simulink model "gait_testing"  (R2024a)
settings: Solver=ode23t  StartTime=0.0  StopTime=8  RelTol=1e-3  AbsTol=1e-3  EnableMultiTasking=on
model workspace (MAT data in the model file):
  A = 0.4
  Length_torso : Simulink.Parameter (value not decoded)
  Lower_limbs : Simulink.Parameter (value not decoded)
  Upper_limbs : Simulink.Parameter (value not decoded)
  Width_torso : Simulink.Parameter (value not decoded)
  f = 1.5
  r_foot : Simulink.Parameter (value not decoded)
  t_leg : Simulink.Parameter (value not decoded)
symbols that are objects in the model workspace (value not decoded): Length_torso, Lower_limbs, t_leg, Upper_limbs, Width_torso
undefined symbols (not defined in the file): P0x, P0z, P1x, P1z, P2x, P2z, X, Y, Z
libraries: sm_lib x88, functionAngles x16, functionAnglesSide x16, nesl_utility x15
(part 4 of 10)

== system gait_testing/Gait Selector/Walk Back Gait - Bezier Curves ==
  t : Inport
  tdur : Inport  Port=2
  change? : Inport  Port=3
  Action Port : ActionPort  InitializeStates=reset  ActionPortLabel=case [ 3 ]:
  Bus Creator : BusCreator  Inputs=12
  Constant{,1..3} (4 alike) : Constant  Value=0
  MATLAB Function : MATLAB Function  TreatAsAtomicUnit=on
  Mod4 : Math  Operator=mod
  Plane Movement : Subsystem
  Plane Movement1 : Subsystem
  Plane Movement2 : Subsystem
  Plane Movement3 : Subsystem
  Plane Movement4 : Subsystem
  Sin-Movement : Subsystem
  Stop when change : Subsystem
  delay and stop when change : Subsystem  mask{delay=0.5}
  delay and stop when change1 : Subsystem  mask{delay=0.25}
  delay and stop when change2 : Subsystem  mask{delay=0.75}
  q : Outport
  wires:
  Constant2/1 -> Bus Creator/12  "sBRs"
  Constant3/1 -> Bus Creator/9  "sBLs"
  Constant1/1 -> Bus Creator/6  "sFRs"
  Constant/1 -> Bus Creator/3  "sFLs"
  Plane Movement3/1(hip) -> Bus Creator/10  "sBR"
  Plane Movement3/2(knee) -> Bus Creator/11  "kBR"
  Plane Movement2/1(hip) -> Bus Creator/7  "sBL"
  Plane Movement2/2(knee) -> Bus Creator/8  "kBL"
  Plane Movement1/2(knee) -> Bus Creator/5  "kFR"
  Plane Movement4/2(knee) -> Bus Creator/2  "kFL"
  Plane Movement1/1(hip) -> Bus Creator/4  "sFR"
  Plane Movement4/1(hip) -> Bus Creator/1  "sFL"
  Bus Creator/1 -> q/1
  Mod4/1 -> Stop when change/3(t_leg)  "t"
  Stop when change/1(t_out) -> Plane Movement4/1(t)
  delay and stop when change2/1(t_leg) -> Plane Movement3/1(t)
  delay and stop when change1/1(t_leg) -> Plane Movement2/1(t)
  MATLAB Function/1(activationTime) -> Stop when change/5(activation time), delay and stop when change2/1(activationTime), delay and stop when change1/1(activationTime), delay and stop when change/1(activationTime)
  delay and stop when change/1(t_leg) -> Plane Movement1/1(t)
  change?/1 -> Stop when change/1(change?), delay and stop when change2/4(Change?), delay and stop when change1/4(Change?), delay and stop when change/4(Change?)
  tdur/1 -> Plane Movement1/2(tdur), delay and stop when change/3(tdur), Plane Movement3/2(tdur), delay and stop when change2/3(tdur), Plane Movement2/2(tdur), delay and stop when change1/3(tdur), Mod4/2, Stop when change/4(tdur), Plane Movement4/2(tdur)
  t/1 -> delay and stop when change2/2(t), delay and stop when change1/2(t), delay and stop when change/2(t), MATLAB Function/1(u), Stop when change/2(t), Mod4/1

== system gait_testing/Gait Selector/Walk Gait - Bezier Curves ==
  t : Inport
  tdur : Inport  Port=2
  Change? : Inport  Port=3
  Action Port : ActionPort  InitializeStates=reset  ActionPortLabel=case [ 1 ]:
  Bus Creator : BusCreator  Inputs=12
  Constant{,1..3} (4 alike) : Constant  Value=0
  MATLAB Function : MATLAB Function  TreatAsAtomicUnit=on
  Mod4 : Math  Operator=mod
  Plane Movement : Subsystem
  Plane Movement1 : Subsystem
  Plane Movement2 : Subsystem
  Plane Movement3 : Subsystem
  Plane Movement4 : Subsystem
  Scope : Scope  NumInputPorts=2
  Sin-Movement : Subsystem
  Stop when change : Subsystem
  delay and stop when change : Subsystem  mask{delay=0.5}
  delay and stop when change1 : Subsystem  mask{delay=0.75}
  delay and stop when change2 : Subsystem  mask{delay=0.25}
  q : Outport
  wires:
  Constant2/1 -> Bus Creator/12  "sBRs"
  Constant3/1 -> Bus Creator/9  "sBLs"
  Constant1/1 -> Bus Creator/6  "sFRs"
  Constant/1 -> Bus Creator/3  "sFLs"
  Mod4/1 -> Stop when change/3(t_leg)  "t"
  tdur/1 -> delay and stop when change2/3(tdur), Plane Movement3/2(tdur), delay and stop when change1/3(tdur), Plane Movement2/2(tdur), Plane Movement1/2(tdur), delay and stop when change/3(tdur), Mod4/2, Stop when change/4(tdur), Plane Movement4/2(tdur)
  t/1 -> Mod4/1, Stop when change/2(t), MATLAB Function/1(u), delay and stop when change2/2(t), delay and stop when change1/2(t), delay and stop when change/2(t)
  Plane Movement3/1(hip) -> Bus Creator/10  "sBR"
  Plane Movement3/2(knee) -> Bus Creator/11  "kBR"
  Plane Movement2/1(hip) -> Bus Creator/7  "sBL"
  Plane Movement2/2(knee) -> Bus Creator/8  "kBL"
  Plane Movement1/2(knee) -> Bus Creator/5  "kFR"
  Plane Movement4/2(knee) -> Scope/1, Bus Creator/2  "kFL"
  Plane Movement1/1(hip) -> Bus Creator/4  "sFR"
  Plane Movement4/1(hip) -> Scope/2, Bus Creator/1  "sFL"
  Bus Creator/1 -> q/1
  MATLAB Function/1(activationTime) -> Stop when change/5(activation time), delay and stop when change2/1(activationTime), delay and stop when change1/1(activationTime), delay and stop when change/1(activationTime)
  delay and stop when change/1(t_leg) -> Plane Movement1/1(t)
  Change?/1 -> delay and stop when change/4(Change?), delay and stop when change1/4(Change?), delay and stop when change2/4(Change?), Stop when change/1(change?)
  Stop when change/1(t_out) -> Plane Movement4/1(t)
  delay and stop when change1/1(t_leg) -> Plane Movement2/1(t)
  delay and stop when change2/1(t_leg) -> Plane Movement3/1(t)

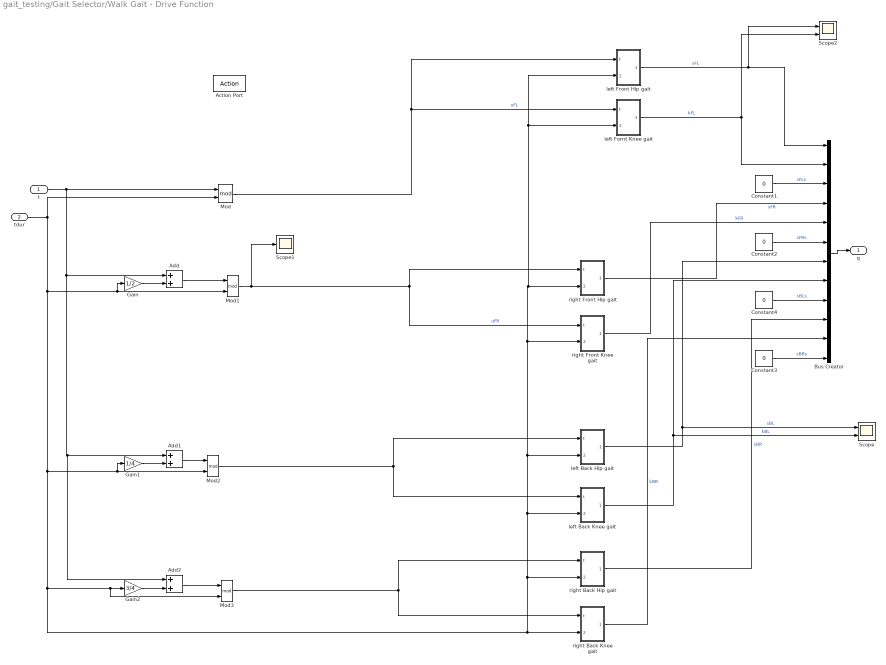
== system gait_testing/Gait Selector/Walk Gait - Drive Function ==
  t : Inport
  tdur : Inport  Port=2
  Action Port : ActionPort  InitializeStates=reset
  Add : Sum
  Add1 : Sum
  Add2 : Sum
  Bus Creator : BusCreator  Inputs=12
  Constant{1..4} (4 alike) : Constant  Value=0
  Gain : Gain  Gain=1/2
  Gain1 : Gain  Gain=1/4
  Gain2 : Gain  Gain=3/4
  Mod{,1..3} (4 alike) : Math  Operator=mod
  Scope : Scope  NumInputPorts=2
  Scope1 : Scope
  Scope2 : Scope  NumInputPorts=2
  left Back Hip gait : Subsystem
  left Back Knee gait : Subsystem
  left Fornt Knee gait : Subsystem
  left Front Hip gait : Subsystem
  right Back Hip gait : Subsystem
  right Back Knee gait : Subsystem
  right Front Hip gait : Subsystem
  right Front Knee gait : Subsystem
  q : Outport
  wires:
  Bus Creator/1 -> q/1
  left Front Hip gait/1(Out1) -> Scope2/1, Bus Creator/1  "sFL"
  right Front Hip gait/1(Out1) -> Bus Creator/4  "sFR"
  left Fornt Knee gait/1(Out1) -> Scope2/2, Bus Creator/2  "kFL"
  right Front Knee gait/1(Out1) -> Bus Creator/5  "kFR"
  Mod/1 -> left Front Hip gait/1(t), left Fornt Knee gait/1(t)  "uFL"
  Mod1/1 -> Scope1/1, right Front Hip gait/1(t), right Front Knee gait/1(t)  "uFR"
  left Back Knee gait/1(Out1) -> Scope/2, Bus Creator/8  "kBL"
  left Back Hip gait/1(Out1) -> Scope/1, Bus Creator/7  "sBL"
  right Back Knee gait/1(Out1) -> Bus Creator/11  "kBR"
  right Back Hip gait/1(Out1) -> Bus Creator/10  "sBR"
  Mod2/1 -> left Back Hip gait/1(t), left Back Knee gait/1(t)
  Mod3/1 -> right Back Knee gait/1(t), right Back Hip gait/1(t)
  t/1 -> Mod/1, Add2/1, Add1/1, Add/1
  Gain2/1 -> Add2/2
  tdur/1 -> Mod/2, left Back Knee gait/2(tdur), left Back Hip gait/2(tdur), right Front Knee gait/2(tdur), right Front Hip gait/2(tdur), left Front Hip gait/2(tdur), left Fornt Knee gait/2(tdur), right Back Hip gait/2(tdur), right Back Knee gait/2(tdur), Gain2/1, Mod3/2, Mod2/2, Gain1/1, Gain/1, Mod1/2
  Add1/1 -> Mod2/1
  Add/1 -> Mod1/1
  Gain/1 -> Add/2
  Gain1/1 -> Add1/2
  Add2/1 -> Mod3/1
  Constant1/1 -> Bus Creator/3  "sFLs"
  Constant3/1 -> Bus Creator/12  "sBRs"
  Constant4/1 -> Bus Creator/9  "sBLs"
  Constant2/1 -> Bus Creator/6  "sFRs"

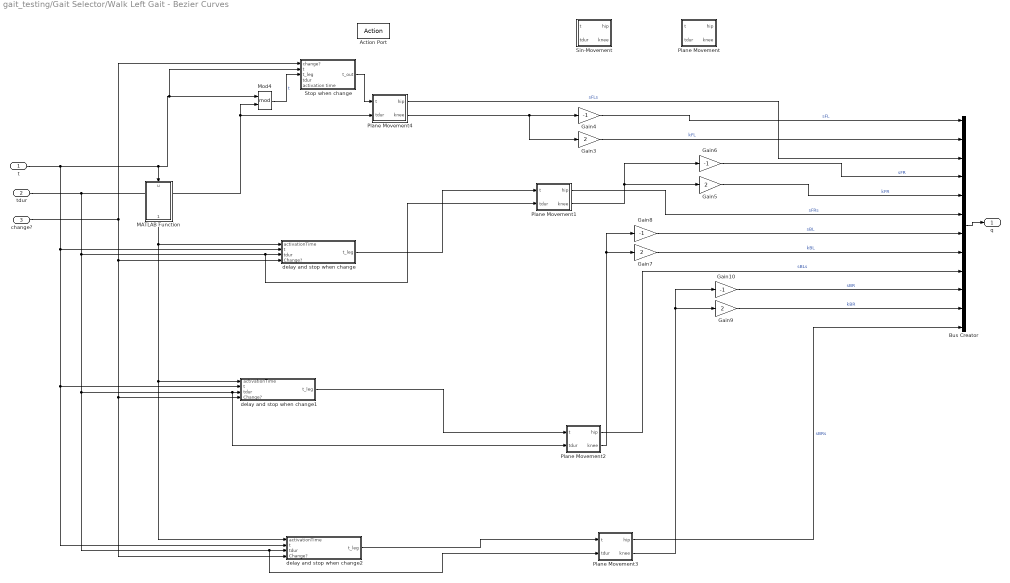
== system gait_testing/Gait Selector/Walk Left Gait - Bezier Curves ==
  t : Inport
  tdur : Inport  Port=2
  change? : Inport  Port=3
  Action Port : ActionPort  InitializeStates=reset  ActionPortLabel=case [ 4 ]:
  Bus Creator : BusCreator  Inputs=12
  Gain{4,6,8,10} (4 alike) : Gain  Gain=-1
  Gain{3,5,7,9} (4 alike) : Gain  Gain=2
  MATLAB Function : MATLAB Function  TreatAsAtomicUnit=on
  Mod4 : Math  Operator=mod
  Plane Movement : Subsystem
  Plane Movement1 : Subsystem
  Plane Movement2 : Subsystem
  Plane Movement3 : Subsystem
  Plane Movement4 : Subsystem
  Sin-Movement : Subsystem
  Stop when change : Subsystem
  delay and stop when change : Subsystem  mask{delay=0.5}
  delay and stop when change1 : Subsystem  mask{delay=0.25}
  delay and stop when change2 : Subsystem  mask{delay=0.75}
  q : Outport
  wires:
  Bus Creator/1 -> q/1
  Plane Movement4/1(hip) -> Bus Creator/3  "sFLs"
  Plane Movement1/1(hip) -> Bus Creator/6  "sFRs"
  Plane Movement4/2(knee) -> Gain3/1, Gain4/1
  Plane Movement1/2(knee) -> Gain6/1, Gain5/1
  Plane Movement2/2(knee) -> Gain7/1, Gain8/1
  Plane Movement2/1(hip) -> Bus Creator/9  "sBLs"
  Plane Movement3/2(knee) -> Gain10/1, Gain9/1
  Plane Movement3/1(hip) -> Bus Creator/12  "sBRs"
  Mod4/1 -> Stop when change/3(t_leg)  "t"
  Gain4/1 -> Bus Creator/1  "sFL"
  Gain5/1 -> Bus Creator/5  "kFR"
  Gain6/1 -> Bus Creator/4  "sFR"
  Gain7/1 -> Bus Creator/8  "kBL"
  Gain8/1 -> Bus Creator/7  "sBL"
  Gain9/1 -> Bus Creator/11  "kBR"
  Gain10/1 -> Bus Creator/10  "sBR"
  Gain3/1 -> Bus Creator/2  "kFL"
  Stop when change/1(t_out) -> Plane Movement4/1(t)
  delay and stop when change2/1(t_leg) -> Plane Movement3/1(t)
  delay and stop when change1/1(t_leg) -> Plane Movement2/1(t)
  delay and stop when change/1(t_leg) -> Plane Movement1/1(t)
  t/1 -> delay and stop when change2/2(t), delay and stop when change1/2(t), delay and stop when change/2(t), Stop when change/2(t), Mod4/1, MATLAB Function/1(u)
  change?/1 -> delay and stop when change2/4(Change?), delay and stop when change1/4(Change?), delay and stop when change/4(Change?), Stop when change/1(change?)
  tdur/1 -> Plane Movement1/2(tdur), delay and stop when change/3(tdur), Plane Movement3/2(tdur), delay and stop when change2/3(tdur), Plane Movement2/2(tdur), delay and stop when change1/3(tdur), Plane Movement4/2(tdur), Mod4/2
  MATLAB Function/1(activationTime) -> delay and stop when change/1(activationTime), delay and stop when change2/1(activationTime), delay and stop when change1/1(activationTime)

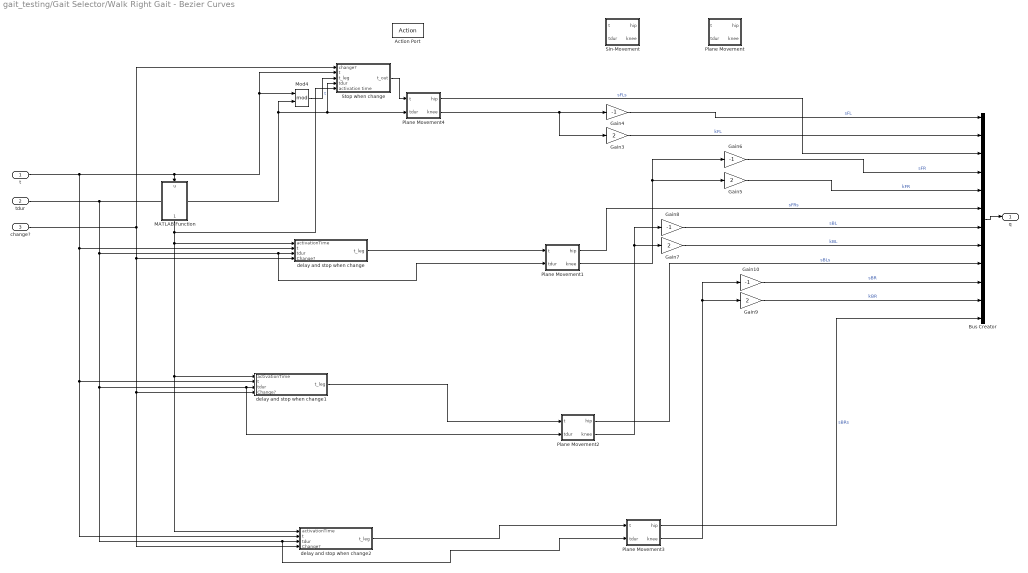
== system gait_testing/Gait Selector/Walk Right Gait - Bezier Curves ==
  t : Inport
  tdur : Inport  Port=2
  change? : Inport  Port=3
  Action Port : ActionPort  InitializeStates=reset  ActionPortLabel=case [ 5 ]:
  Bus Creator : BusCreator  Inputs=12
  Gain{4,6,8,10} (4 alike) : Gain  Gain=-1
  Gain{3,5,7,9} (4 alike) : Gain  Gain=2
  MATLAB Function : MATLAB Function  TreatAsAtomicUnit=on
  Mod4 : Math  Operator=mod
  Plane Movement : Subsystem
  Plane Movement1 : Subsystem
  Plane Movement2 : Subsystem
  Plane Movement3 : Subsystem
  Plane Movement4 : Subsystem
  Sin-Movement : Subsystem
  Stop when change : Subsystem
  delay and stop when change : Subsystem  mask{delay=0.5}
  delay and stop when change1 : Subsystem  mask{delay=0.25}
  delay and stop when change2 : Subsystem  mask{delay=0.75}
  q : Outport
  wires:
  Gain3/1 -> Bus Creator/2  "kFL"
  Gain10/1 -> Bus Creator/10  "sBR"
  Gain9/1 -> Bus Creator/11  "kBR"
  Gain8/1 -> Bus Creator/7  "sBL"
  Gain7/1 -> Bus Creator/8  "kBL"
  Gain6/1 -> Bus Creator/4  "sFR"
  Gain5/1 -> Bus Creator/5  "kFR"
  Gain4/1 -> Bus Creator/1  "sFL"
  Mod4/1 -> Stop when change/3(t_leg)  "t"
  Plane Movement3/1(hip) -> Bus Creator/12  "sBRs"
  Plane Movement3/2(knee) -> Gain9/1, Gain10/1
  Plane Movement2/1(hip) -> Bus Creator/9  "sBLs"
  Plane Movement2/2(knee) -> Gain8/1, Gain7/1
  Plane Movement1/2(knee) -> Gain5/1, Gain6/1
  Plane Movement4/2(knee) -> Gain4/1, Gain3/1
  Plane Movement1/1(hip) -> Bus Creator/6  "sFRs"
  Plane Movement4/1(hip) -> Bus Creator/3  "sFLs"
  Bus Creator/1 -> q/1
  Stop when change/1(t_out) -> Plane Movement4/1(t)
  delay and stop when change2/1(t_leg) -> Plane Movement3/1(t)
  delay and stop when change1/1(t_leg) -> Plane Movement2/1(t)
  delay and stop when change/1(t_leg) -> Plane Movement1/1(t)
  t/1 -> delay and stop when change2/2(t), delay and stop when change1/2(t), delay and stop when change/2(t), Stop when change/2(t), Mod4/1, MATLAB Function/1(u)
  change?/1 -> delay and stop when change2/4(Change?), delay and stop when change1/4(Change?), delay and stop when change/4(Change?), Stop when change/1(change?)
  tdur/1 -> Plane Movement1/2(tdur), delay and stop when change/3(tdur), Plane Movement3/2(tdur), delay and stop when change2/3(tdur), Plane Movement2/2(tdur), delay and stop when change1/3(tdur), Mod4/2, Stop when change/4(tdur), Plane Movement4/2(tdur)
  MATLAB Function/1(activationTime) -> Stop when change/5(activation time), delay and stop when change/1(activationTime), delay and stop when change2/1(activationTime), delay and stop when change1/1(activationTime)

== system gait_testing/Gait Selector/Stand Still/Plane Movement ==
  t : Inport
  tdur : Inport  Port=2
  Constant : Constant  Value=P0x
  Constant1 : Constant  Value=P0z
  Constant2 : Constant  Value=P1z
  Constant3 : Constant  Value=P1x
  Constant4 : Constant  Value=P2x
  Constant5 : Constant  Value=P2z
  Constant6 : Constant  Value=P3x
  Constant7 : Constant  Value=P3z
  Gain : Gain  Gain=180/pi
  Gain1 : Gain  Gain=-180/pi
  Length lower Limb : Constant  Value=Lower_limbs
  Length upper Limb : Constant  Value=Upper_limbs
  MATLAB Function1 : MATLAB Function  TreatAsAtomicUnit=on
  MATLAB Function2 : MATLAB Function  TreatAsAtomicUnit=on
  Scope : Scope  NumInputPorts=2
  Subsystem1 : Subsystem  Commented=on
  hip : Outport
  knee : Outport  Port=2
  wires:
  MATLAB Function2/2(y) -> MATLAB Function1/2(y), Scope/2
  MATLAB Function2/1(x) -> Scope/1, MATLAB Function1/1(x)
  MATLAB Function1/2(theta2) -> Gain1/1  "knee"
  tdur/1 -> MATLAB Function2/2(Tdur)
  MATLAB Function1/1(theta1) -> Gain/1  "hip"
  t/1 -> MATLAB Function2/1(t)
  Length upper Limb/1 -> MATLAB Function1/3(L1)
  Length lower Limb/1 -> MATLAB Function1/4(L2)
  Gain1/1 -> knee/1
  Gain/1 -> hip/1
  Constant/1 -> MATLAB Function2/3(P0x)
  Constant1/1 -> MATLAB Function2/4(P0z)
  Constant3/1 -> MATLAB Function2/5(P1x)
  Constant2/1 -> MATLAB Function2/6(P1z)
  Constant4/1 -> MATLAB Function2/7(P2x)
  Constant5/1 -> MATLAB Function2/8(P2z)
  Constant6/1 -> MATLAB Function2/9(P3x)
  Constant7/1 -> MATLAB Function2/10(P3z)

== system gait_testing/Gait Selector/Stand Still/Plane Movement1 ==
  t : Inport
  tdur : Inport  Port=2
  Constant : Constant  Value=P3x
  Constant1 : Constant  Value=P3z
  Gain : Gain  Gain=180/pi
  Gain1 : Gain  Gain=-180/pi
  Length lower Limb : Constant  Value=Lower_limbs
  Length upper Limb : Constant  Value=Upper_limbs
  MATLAB : functionAngles/MATLAB  SystemSampleTime=-1  VariantActivationTime=update diagram  AllowFlexibleInterface=on  Latency=0  AutoFrameSizeCalculation=off
  Subsystem1 : Subsystem  Commented=on
  hip : Outport
  knee : Outport  Port=2
  wires:
  MATLAB/2 -> Gain1/1  "knee"
  tdur/1 -> ?
  MATLAB/1 -> Gain/1  "hip"
  t/1 -> ?
  Length upper Limb/1 -> MATLAB/3
  Length lower Limb/1 -> MATLAB/4
  Gain1/1 -> knee/1
  Gain/1 -> hip/1
  Constant/1 -> MATLAB/1
  Constant1/1 -> MATLAB/2

== system gait_testing/Gait Selector/Stand Still/Plane Movement2 ==
  t : Inport
  tdur : Inport  Port=2
  Constant : Constant  Value=P3x
  Constant1 : Constant  Value=P3z
  Gain : Gain  Gain=180/pi
  Gain1 : Gain  Gain=-180/pi
  Length lower Limb : Constant  Value=Lower_limbs
  Length upper Limb : Constant  Value=Upper_limbs
  MATLAB : functionAngles/MATLAB  SystemSampleTime=-1  VariantActivationTime=update diagram  AllowFlexibleInterface=on  Latency=0  AutoFrameSizeCalculation=off
  Subsystem1 : Subsystem  Commented=on
  hip : Outport
  knee : Outport  Port=2
  wires:
  Constant1/1 -> MATLAB/2
  Constant/1 -> MATLAB/1
  Gain/1 -> hip/1
  Gain1/1 -> knee/1
  Length lower Limb/1 -> MATLAB/4
  Length upper Limb/1 -> MATLAB/3
  t/1 -> ?
  MATLAB/1 -> Gain/1  "hip"
  tdur/1 -> ?
  MATLAB/2 -> Gain1/1  "knee"

== system gait_testing/Gait Selector/Stand Still/Plane Movement3 ==
  t : Inport
  tdur : Inport  Port=2
  Constant : Constant  Value=P3x
  Constant1 : Constant  Value=P3z
  Gain : Gain  Gain=180/pi
  Gain1 : Gain  Gain=-180/pi
  Length lower Limb : Constant  Value=Lower_limbs
  Length upper Limb : Constant  Value=Upper_limbs
  MATLAB : functionAngles/MATLAB  SystemSampleTime=-1  VariantActivationTime=update diagram  AllowFlexibleInterface=on  Latency=0  AutoFrameSizeCalculation=off
  Subsystem1 : Subsystem  Commented=on
  hip : Outport
  knee : Outport  Port=2
  wires:
  MATLAB/2 -> Gain1/1  "knee"
  tdur/1 -> ?
  MATLAB/1 -> Gain/1  "hip"
  t/1 -> ?
  Length upper Limb/1 -> MATLAB/3
  Length lower Limb/1 -> MATLAB/4
  Gain1/1 -> knee/1
  Gain/1 -> hip/1
  Constant/1 -> MATLAB/1
  Constant1/1 -> MATLAB/2

== system gait_testing/Gait Selector/Stand Still/Plane Movement4 ==
  t : Inport
  tdur : Inport  Port=2
  Constant : Constant  Value=P3x
  Constant1 : Constant  Value=P3z
  Gain : Gain  Gain=180/pi
  Gain1 : Gain  Gain=-180/pi
  Length lower Limb : Constant  Value=Lower_limbs
  Length upper Limb : Constant  Value=Upper_limbs
  MATLAB : functionAngles/MATLAB  SystemSampleTime=-1  VariantActivationTime=update diagram  AllowFlexibleInterface=on  Latency=0  AutoFrameSizeCalculation=off
  Subsystem1 : Subsystem  Commented=on
  hip : Outport
  knee : Outport  Port=2
  wires:
  Constant1/1 -> MATLAB/2
  Constant/1 -> MATLAB/1
  Gain/1 -> hip/1
  Gain1/1 -> knee/1
  Length lower Limb/1 -> MATLAB/4
  Length upper Limb/1 -> MATLAB/3
  t/1 -> ?
  MATLAB/1 -> Gain/1  "hip"
  tdur/1 -> ?
  MATLAB/2 -> Gain1/1  "knee"

== system gait_testing/Gait Selector/Stand Still/Sin-Movement ==
  t : Inport
  tdur : Inport  Port=2
  Constant : Constant  Value=P0x
  Constant1 : Constant  Value=P0z
  Constant2 : Constant  Value=P1z
  Constant3 : Constant  Value=P1x
  Constant4 : Constant  Value=P2x
  Constant5 : Constant  Value=P2z
  Constant6 : Constant  Value=P3x
  Constant7 : Constant  Value=P3z
  Gain : Gain  Gain=180/pi
  Gain1 : Gain  Gain=-180/pi
  Length lower Limb : Constant  Value=Lower_limbs
  Length upper Limb : Constant  Value=Upper_limbs
  MATLAB Function : MATLAB Function  TreatAsAtomicUnit=on
  MATLAB Function1 : MATLAB Function  TreatAsAtomicUnit=on
  Scope : Scope  NumInputPorts=2
  Subsystem1 : Subsystem  Commented=on
  hip : Outport
  knee : Outport  Port=2
  wires:
  MATLAB Function/2(y) -> MATLAB Function1/2(y), Scope/2
  MATLAB Function/1(x) -> MATLAB Function1/1(x), Scope/1
  MATLAB Function1/2(theta2) -> Gain1/1  "knee"
  tdur/1 -> MATLAB Function/2(Tdur)
  MATLAB Function1/1(theta1) -> Gain/1  "hip"
  t/1 -> MATLAB Function/1(t)
  Length upper Limb/1 -> MATLAB Function1/3(L1)
  Length lower Limb/1 -> MATLAB Function1/4(L2)
  Gain1/1 -> knee/1
  Gain/1 -> hip/1
  Constant/1 -> MATLAB Function/3(P0x)
  Constant1/1 -> MATLAB Function/4(P0z)
  Constant3/1 -> MATLAB Function/5(P1x)
  Constant2/1 -> MATLAB Function/6(P1z)
  Constant4/1 -> MATLAB Function/7(P2x)
  Constant5/1 -> MATLAB Function/8(P2z)
  Constant6/1 -> MATLAB Function/9(P3x)
  Constant7/1 -> MATLAB Function/10(P3z)

== system gait_testing/Gait Selector/Trot Gait - Bezier Curves/Plane Movement ==
  t : Inport
  tdur : Inport  Port=2
  Constant : Constant  Value=P0x
  Constant1 : Constant  Value=P0z
  Constant2 : Constant  Value=P1z
  Constant3 : Constant  Value=P1x
  Constant4 : Constant  Value=P2x
  Constant5 : Constant  Value=P2z
  Constant6 : Constant  Value=P3x
  Constant7 : Constant  Value=P3z
  Gain : Gain  Gain=180/pi
  Gain1 : Gain  Gain=-180/pi
  Length lower Limb : Constant  Value=Lower_limbs
  Length upper Limb : Constant  Value=Upper_limbs
  MATLAB Function1 : MATLAB Function  TreatAsAtomicUnit=on
  MATLAB Function2 : MATLAB Function  TreatAsAtomicUnit=on
  Scope : Scope  NumInputPorts=2
  Subsystem1 : Subsystem  Commented=on
  hip : Outport
  knee : Outport  Port=2
  wires:
  MATLAB Function2/2(y) -> MATLAB Function1/2(y), Scope/2
  MATLAB Function2/1(x) -> Scope/1, MATLAB Function1/1(x)
  MATLAB Function1/2(theta2) -> Gain1/1  "knee"
  tdur/1 -> MATLAB Function2/2(Tdur)
  MATLAB Function1/1(theta1) -> Gain/1  "hip"
  t/1 -> MATLAB Function2/1(t)
  Length upper Limb/1 -> MATLAB Function1/3(L1)
  Length lower Limb/1 -> MATLAB Function1/4(L2)
  Gain1/1 -> knee/1
  Gain/1 -> hip/1
  Constant/1 -> MATLAB Function2/3(P0x)
  Constant1/1 -> MATLAB Function2/4(P0z)
  Constant3/1 -> MATLAB Function2/5(P1x)
  Constant2/1 -> MATLAB Function2/6(P1z)
  Constant4/1 -> MATLAB Function2/7(P2x)
  Constant5/1 -> MATLAB Function2/8(P2z)
  Constant6/1 -> MATLAB Function2/9(P3x)
  Constant7/1 -> MATLAB Function2/10(P3z)

== system gait_testing/Gait Selector/Trot Gait - Bezier Curves/Plane Movement1 ==
  t : Inport
  tdur : Inport  Port=2
  Constant : Constant  Value=P0x
  Constant1 : Constant  Value=P0z
  Constant2 : Constant  Value=P1z
  Constant3 : Constant  Value=P1x
  Constant4 : Constant  Value=P2x
  Constant5 : Constant  Value=P2z
  Constant6 : Constant  Value=P3x
  Constant7 : Constant  Value=P3z
  Gain : Gain  Gain=180/pi
  Gain1 : Gain  Gain=-180/pi
  Length lower Limb : Constant  Value=Lower_limbs
  Length upper Limb : Constant  Value=Upper_limbs
  MATLAB : functionAngles/MATLAB  SystemSampleTime=-1  VariantActivationTime=update diagram  AllowFlexibleInterface=on  Latency=0  AutoFrameSizeCalculation=off
  MATLAB Function2 : MATLAB Function  TreatAsAtomicUnit=on
  Scope : Scope  NumInputPorts=2
  Subsystem1 : Subsystem  Commented=on
  hip : Outport
  knee : Outport  Port=2
  wires:
  Constant7/1 -> MATLAB Function2/10(P3z)
  Constant6/1 -> MATLAB Function2/9(P3x)
  Constant5/1 -> MATLAB Function2/8(P2z)
  Constant4/1 -> MATLAB Function2/7(P2x)
  Constant2/1 -> MATLAB Function2/6(P1z)
  Constant3/1 -> MATLAB Function2/5(P1x)
  Constant1/1 -> MATLAB Function2/4(P0z)
  Constant/1 -> MATLAB Function2/3(P0x)
  Gain/1 -> hip/1
  Gain1/1 -> knee/1
  Length lower Limb/1 -> MATLAB/4
  Length upper Limb/1 -> MATLAB/3
  t/1 -> MATLAB Function2/1(t)
  MATLAB/1 -> Gain/1  "hip"
  tdur/1 -> MATLAB Function2/2(Tdur)
  MATLAB/2 -> Gain1/1  "knee"
  MATLAB Function2/1(x) -> MATLAB/1, Scope/1
  MATLAB Function2/2(y) -> MATLAB/2, Scope/2

== system gait_testing/Gait Selector/Trot Gait - Bezier Curves/Plane Movement2 ==
  t : Inport
  tdur : Inport  Port=2
  Constant : Constant  Value=P0x
  Constant1 : Constant  Value=P0z
  Constant2 : Constant  Value=P1z
  Constant3 : Constant  Value=P1x
  Constant4 : Constant  Value=P2x
  Constant5 : Constant  Value=P2z
  Constant6 : Constant  Value=P3x
  Constant7 : Constant  Value=P3z
  Gain : Gain  Gain=180/pi
  Gain1 : Gain  Gain=-180/pi
  Length lower Limb : Constant  Value=Lower_limbs
  Length upper Limb : Constant  Value=Upper_limbs
  MATLAB : functionAngles/MATLAB  SystemSampleTime=-1  VariantActivationTime=update diagram  AllowFlexibleInterface=on  Latency=0  AutoFrameSizeCalculation=off
  MATLAB Function2 : MATLAB Function  TreatAsAtomicUnit=on
  Scope : Scope  NumInputPorts=2
  Subsystem1 : Subsystem  Commented=on
  hip : Outport
  knee : Outport  Port=2
  wires:
  Constant7/1 -> MATLAB Function2/10(P3z)
  Constant6/1 -> MATLAB Function2/9(P3x)
  Constant5/1 -> MATLAB Function2/8(P2z)
  Constant4/1 -> MATLAB Function2/7(P2x)
  Constant2/1 -> MATLAB Function2/6(P1z)
  Constant3/1 -> MATLAB Function2/5(P1x)
  Constant1/1 -> MATLAB Function2/4(P0z)
  Constant/1 -> MATLAB Function2/3(P0x)
  Gain/1 -> hip/1
  Gain1/1 -> knee/1
  Length lower Limb/1 -> MATLAB/4
  Length upper Limb/1 -> MATLAB/3
  t/1 -> MATLAB Function2/1(t)
  MATLAB/1 -> Gain/1  "hip"
  tdur/1 -> MATLAB Function2/2(Tdur)
  MATLAB/2 -> Gain1/1  "knee"
  MATLAB Function2/1(x) -> MATLAB/1, Scope/1
  MATLAB Function2/2(y) -> MATLAB/2, Scope/2

== system gait_testing/Gait Selector/Trot Gait - Bezier Curves/Plane Movement3 ==
  t : Inport
  tdur : Inport  Port=2
  Constant : Constant  Value=P0x
  Constant1 : Constant  Value=P0z
  Constant2 : Constant  Value=P1z
  Constant3 : Constant  Value=P1x
  Constant4 : Constant  Value=P2x
  Constant5 : Constant  Value=P2z
  Constant6 : Constant  Value=P3x
  Constant7 : Constant  Value=P3z
  Gain : Gain  Gain=180/pi
  Gain1 : Gain  Gain=-180/pi
  Length lower Limb : Constant  Value=Lower_limbs
  Length upper Limb : Constant  Value=Upper_limbs
  MATLAB : functionAngles/MATLAB  SystemSampleTime=-1  VariantActivationTime=update diagram  AllowFlexibleInterface=on  Latency=0  AutoFrameSizeCalculation=off
  MATLAB Function2 : MATLAB Function  TreatAsAtomicUnit=on
  Scope : Scope  NumInputPorts=2
  Subsystem1 : Subsystem  Commented=on
  hip : Outport
  knee : Outport  Port=2
  wires:
  MATLAB Function2/2(y) -> MATLAB/2, Scope/2
  MATLAB Function2/1(x) -> MATLAB/1, Scope/1
  MATLAB/2 -> Gain1/1  "knee"
  tdur/1 -> MATLAB Function2/2(Tdur)
  MATLAB/1 -> Gain/1  "hip"
  t/1 -> MATLAB Function2/1(t)
  Length upper Limb/1 -> MATLAB/3
  Length lower Limb/1 -> MATLAB/4
  Gain1/1 -> knee/1
  Gain/1 -> hip/1
  Constant/1 -> MATLAB Function2/3(P0x)
  Constant1/1 -> MATLAB Function2/4(P0z)
  Constant3/1 -> MATLAB Function2/5(P1x)
  Constant2/1 -> MATLAB Function2/6(P1z)
  Constant4/1 -> MATLAB Function2/7(P2x)
  Constant5/1 -> MATLAB Function2/8(P2z)
  Constant6/1 -> MATLAB Function2/9(P3x)
  Constant7/1 -> MATLAB Function2/10(P3z)

== system gait_testing/Gait Selector/Trot Gait - Bezier Curves/Plane Movement4 ==
  t : Inport
  tdur : Inport  Port=2
  Constant : Constant  Value=P0x
  Constant1 : Constant  Value=P0z
  Constant2 : Constant  Value=P1z
  Constant3 : Constant  Value=P1x
  Constant4 : Constant  Value=P2x
  Constant5 : Constant  Value=P2z
  Constant6 : Constant  Value=P3x
  Constant7 : Constant  Value=P3z
  Gain : Gain  Gain=180/pi
  Gain1 : Gain  Gain=-180/pi
  Length lower Limb : Constant  Value=Lower_limbs
  Length upper Limb : Constant  Value=Upper_limbs
  MATLAB : functionAngles/MATLAB  SystemSampleTime=-1  VariantActivationTime=update diagram  AllowFlexibleInterface=on  Latency=0  AutoFrameSizeCalculation=off
  MATLAB Function2 : MATLAB Function  TreatAsAtomicUnit=on
  Scope : Scope  NumInputPorts=2
  Subsystem1 : Subsystem  Commented=on
  hip : Outport
  knee : Outport  Port=2
  wires:
  Constant7/1 -> MATLAB Function2/10(P3z)
  Constant6/1 -> MATLAB Function2/9(P3x)
  Constant5/1 -> MATLAB Function2/8(P2z)
  Constant4/1 -> MATLAB Function2/7(P2x)
  Constant2/1 -> MATLAB Function2/6(P1z)
  Constant3/1 -> MATLAB Function2/5(P1x)
  Constant1/1 -> MATLAB Function2/4(P0z)
  Constant/1 -> MATLAB Function2/3(P0x)
  Gain/1 -> hip/1
  Gain1/1 -> knee/1
  Length lower Limb/1 -> MATLAB/4
  Length upper Limb/1 -> MATLAB/3
  t/1 -> MATLAB Function2/1(t)
  MATLAB/1 -> Gain/1  "hip"
  tdur/1 -> MATLAB Function2/2(Tdur)
  MATLAB/2 -> Gain1/1  "knee"
  MATLAB Function2/1(x) -> MATLAB/1, Scope/1
  MATLAB Function2/2(y) -> MATLAB/2, Scope/2

== system gait_testing/Gait Selector/Trot Gait - Bezier Curves/Sin-Movement ==
  t : Inport
  tdur : Inport  Port=2
  Constant : Constant  Value=P0x
  Constant1 : Constant  Value=P0z
  Constant2 : Constant  Value=P1z
  Constant3 : Constant  Value=P1x
  Constant4 : Constant  Value=P2x
  Constant5 : Constant  Value=P2z
  Constant6 : Constant  Value=P3x
  Constant7 : Constant  Value=P3z
  Gain : Gain  Gain=180/pi
  Gain1 : Gain  Gain=-180/pi
  Length lower Limb : Constant  Value=Lower_limbs
  Length upper Limb : Constant  Value=Upper_limbs
  MATLAB Function : MATLAB Function  TreatAsAtomicUnit=on
  MATLAB Function1 : MATLAB Function  TreatAsAtomicUnit=on
  Scope : Scope  NumInputPorts=2
  Subsystem1 : Subsystem  Commented=on
  hip : Outport
  knee : Outport  Port=2
  wires:
  MATLAB Function/2(y) -> MATLAB Function1/2(y), Scope/2
  MATLAB Function/1(x) -> MATLAB Function1/1(x), Scope/1
  MATLAB Function1/2(theta2) -> Gain1/1  "knee"
  tdur/1 -> MATLAB Function/2(Tdur)
  MATLAB Function1/1(theta1) -> Gain/1  "hip"
  t/1 -> MATLAB Function/1(t)
  Length upper Limb/1 -> MATLAB Function1/3(L1)
  Length lower Limb/1 -> MATLAB Function1/4(L2)
  Gain1/1 -> knee/1
  Gain/1 -> hip/1
  Constant/1 -> MATLAB Function/3(P0x)
  Constant1/1 -> MATLAB Function/4(P0z)
  Constant3/1 -> MATLAB Function/5(P1x)
  Constant2/1 -> MATLAB Function/6(P1z)
  Constant4/1 -> MATLAB Function/7(P2x)
  Constant5/1 -> MATLAB Function/8(P2z)
  Constant6/1 -> MATLAB Function/9(P3x)
  Constant7/1 -> MATLAB Function/10(P3z)

== system gait_testing/Gait Selector/Trot Gait - Bezier Curves/Stop when change ==
  change? : Inport
  t : Inport  Port=2
  t_leg : Inport  Port=3
  tdur : Inport  Port=4
  activation time : Inport  Port=5
  AND : Logic  IconShape=distinctive  AllPortsSameDT=off  OutDataTypeStr=boolean
  Add : Sum  Inputs=+-
  Add2 : Sum  Inputs=+-
  Constant1 : Constant  Value=0
  Constant2 : Constant  Value=0
  OR : Logic  Operator=OR  IconShape=distinctive  AllPortsSameDT=off  OutDataTypeStr=boolean
  Relational Operator : RelationalOperator  Operator=<  OutDataTypeStr=boolean  RndMeth=Simplest  InputSameDT=off
  Relational Operator1 : RelationalOperator  Operator=<=  OutDataTypeStr=boolean  RndMeth=Simplest  InputSameDT=off
  Relational Operator2 : RelationalOperator  Operator===  OutDataTypeStr=boolean  RndMeth=Simplest  InputSameDT=off
  Relational Operator3 : RelationalOperator  Operator=>  OutDataTypeStr=boolean  RndMeth=Simplest  InputSameDT=off
  Switch : Switch  Criteria=u2 > Threshold  SaturateOnIntegerOverflow=off  InputSameDT=off
  Switch Case1 : SwitchCase  ShowDefaultCase=off
  Switch1 : Switch  Criteria=u2 > Threshold  SaturateOnIntegerOverflow=off  InputSameDT=off
  Triggered Subsystem : Subsystem  TreatAsAtomicUnit=on
  Unit Delay : UnitDelay  SampleTime=-1  HasFrameUpgradeWarning=on
  t_out : Outport
  wires:
  t_leg/1 -> Switch/3, Switch1/3, Unit Delay/1, Relational Operator/1
  Add2/1 -> Relational Operator1/1
  change?/1 -> Switch Case1/1
  Switch Case1/1 -> Triggered Subsystem/Action
  AND/1 -> Switch1/2
  Unit Delay/1 -> Relational Operator/2
  Switch1/1 -> Relational Operator2/1, Switch/1
  Relational Operator1/1 -> AND/1
  Constant2/1 -> Relational Operator2/2
  Triggered Subsystem/1(Change Time) -> Add2/2
  Relational Operator/1 -> OR/1
  tdur/1 -> Relational Operator1/2
  Relational Operator2/1 -> OR/2
  OR/1 -> AND/2
  Constant1/1 -> Switch1/1
  t/1 -> Add2/1, Add/1, Triggered Subsystem/1(t)
  Relational Operator3/1 -> Switch/2
  Switch/1 -> t_out/1
  Add/1 -> Relational Operator3/1
  activation time/1 -> Add/2

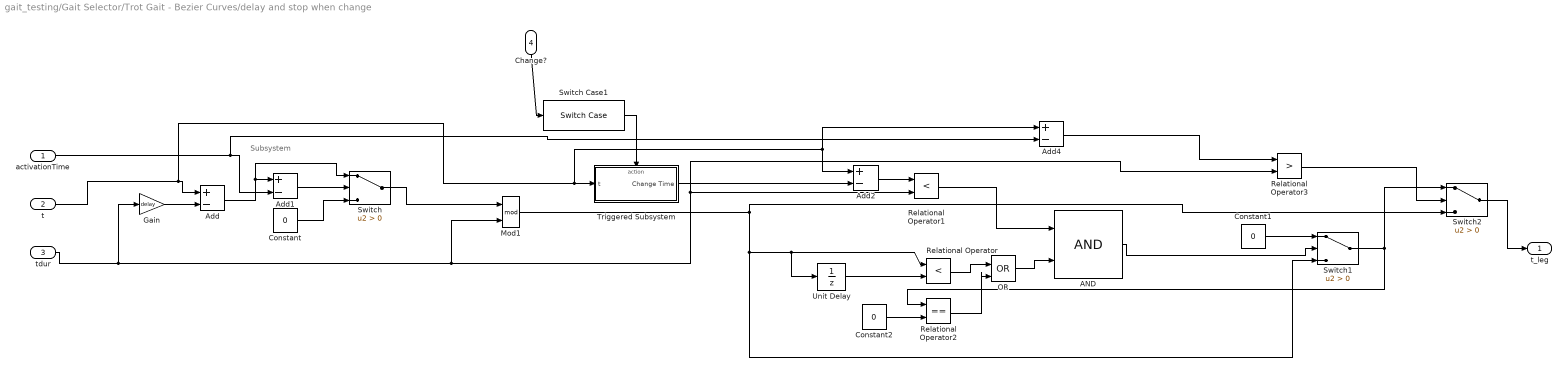
== system gait_testing/Gait Selector/Trot Gait - Bezier Curves/delay and stop when change ==
  note: Subsystem
  activationTime : Inport
  t : Inport  Port=2
  tdur : Inport  Port=3
  Change? : Inport  Port=4
  AND : Logic  IconShape=distinctive  AllPortsSameDT=off  OutDataTypeStr=boolean
  Add{,1..2,4} (4 alike) : Sum  Inputs=+-
  Constant : Constant  Value=0
  Constant1 : Constant  Value=0
  Constant2 : Constant  Value=0
  Gain : Gain  Gain=delay
  Mod1 : Math  Operator=mod
  OR : Logic  Operator=OR  IconShape=distinctive  AllPortsSameDT=off  OutDataTypeStr=boolean
  Relational Operator : RelationalOperator  Operator=<  OutDataTypeStr=boolean  RndMeth=Simplest  InputSameDT=off
  Relational Operator1 : RelationalOperator  Operator=<  OutDataTypeStr=boolean  RndMeth=Simplest  InputSameDT=off
  Relational Operator2 : RelationalOperator  Operator===  OutDataTypeStr=boolean  RndMeth=Simplest  InputSameDT=off
  Relational Operator3 : RelationalOperator  Operator=>  OutDataTypeStr=boolean  RndMeth=Simplest  InputSameDT=off
  Switch : Switch  Criteria=u2 > Threshold  SaturateOnIntegerOverflow=off  InputSameDT=off
  Switch Case1 : SwitchCase  ShowDefaultCase=off
  Switch1 : Switch  Criteria=u2 > Threshold  SaturateOnIntegerOverflow=off  InputSameDT=off
  Switch2 : Switch  Criteria=u2 > Threshold  SaturateOnIntegerOverflow=off  InputSameDT=off
  Triggered Subsystem : Subsystem  TreatAsAtomicUnit=on
  Unit Delay : UnitDelay  SampleTime=-1  HasFrameUpgradeWarning=on
  t_leg : Outport
  wires:
  Switch/1 -> Mod1/1
  Gain/1 -> Add/2
  t/1 -> Add2/1, Add4/1, Triggered Subsystem/1(t), Add/1
  Constant/1 -> Switch/3
  Add1/1 -> Switch/2
  activationTime/1 -> Add4/2, Add1/2
  Add/1 -> Switch/1, Add1/1
  Switch Case1/1 -> Triggered Subsystem/Action
  Relational Operator1/1 -> AND/1
  Constant1/1 -> Switch1/1
  Relational Operator/1 -> OR/1
  Change?/1 -> Switch Case1/1
  Unit Delay/1 -> Relational Operator/2
  AND/1 -> Switch1/2
  Switch1/1 -> Switch2/1, Relational Operator2/1
  Mod1/1 -> Switch2/3, Switch1/3, Unit Delay/1, Relational Operator/1
  Triggered Subsystem/1(Change Time) -> Add2/2
  Add2/1 -> Relational Operator1/1
  Relational Operator2/1 -> OR/2
  Constant2/1 -> Relational Operator2/2
  OR/1 -> AND/2
  Switch2/1 -> t_leg/1
  Relational Operator3/1 -> Switch2/2
  tdur/1 -> Gain/1, Mod1/2, Relational Operator3/2, Relational Operator1/2
  Add4/1 -> Relational Operator3/1

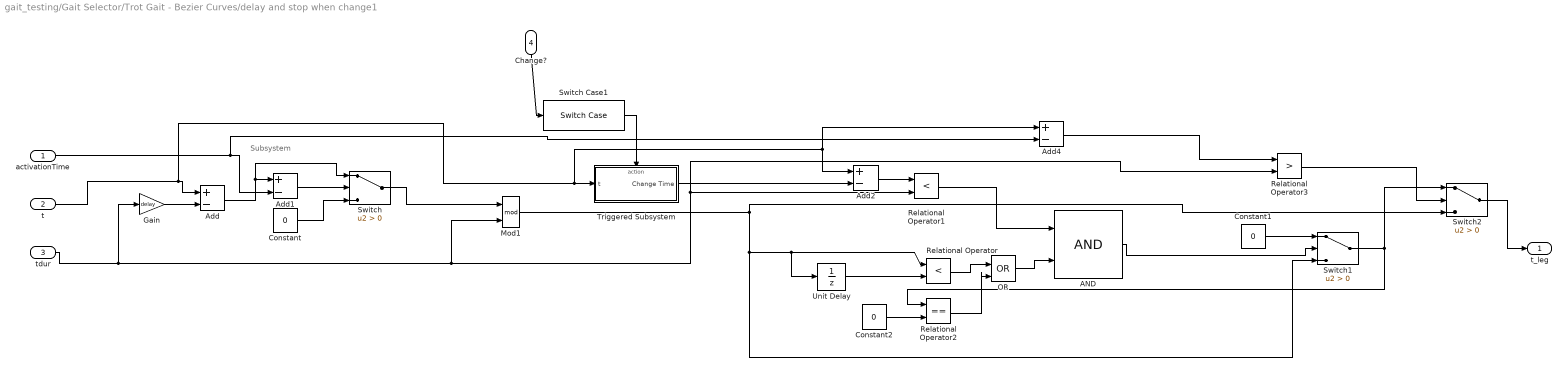
== system gait_testing/Gait Selector/Trot Gait - Bezier Curves/delay and stop when change1 ==
  note: Subsystem
  activationTime : Inport
  t : Inport  Port=2
  tdur : Inport  Port=3
  Change? : Inport  Port=4
  AND : Logic  IconShape=distinctive  AllPortsSameDT=off  OutDataTypeStr=boolean
  Add{,1..2,4} (4 alike) : Sum  Inputs=+-
  Constant : Constant  Value=0
  Constant1 : Constant  Value=0
  Constant2 : Constant  Value=0
  Gain : Gain  Gain=delay
  Mod1 : Math  Operator=mod
  OR : Logic  Operator=OR  IconShape=distinctive  AllPortsSameDT=off  OutDataTypeStr=boolean
  Relational Operator : RelationalOperator  Operator=<  OutDataTypeStr=boolean  RndMeth=Simplest  InputSameDT=off
  Relational Operator1 : RelationalOperator  Operator=<  OutDataTypeStr=boolean  RndMeth=Simplest  InputSameDT=off
  Relational Operator2 : RelationalOperator  Operator===  OutDataTypeStr=boolean  RndMeth=Simplest  InputSameDT=off
  Relational Operator3 : RelationalOperator  Operator=>  OutDataTypeStr=boolean  RndMeth=Simplest  InputSameDT=off
  Switch : Switch  Criteria=u2 > Threshold  SaturateOnIntegerOverflow=off  InputSameDT=off
  Switch Case1 : SwitchCase  ShowDefaultCase=off
  Switch1 : Switch  Criteria=u2 > Threshold  SaturateOnIntegerOverflow=off  InputSameDT=off
  Switch2 : Switch  Criteria=u2 > Threshold  SaturateOnIntegerOverflow=off  InputSameDT=off
  Triggered Subsystem : Subsystem  TreatAsAtomicUnit=on
  Unit Delay : UnitDelay  SampleTime=-1  HasFrameUpgradeWarning=on
  t_leg : Outport
  wires:
  Switch/1 -> Mod1/1
  Gain/1 -> Add/2
  t/1 -> Add2/1, Add4/1, Triggered Subsystem/1(t), Add/1
  Constant/1 -> Switch/3
  Add1/1 -> Switch/2
  activationTime/1 -> Add4/2, Add1/2
  Add/1 -> Switch/1, Add1/1
  Switch Case1/1 -> Triggered Subsystem/Action
  Relational Operator1/1 -> AND/1
  Constant1/1 -> Switch1/1
  Relational Operator/1 -> OR/1
  Change?/1 -> Switch Case1/1
  Unit Delay/1 -> Relational Operator/2
  AND/1 -> Switch1/2
  Switch1/1 -> Switch2/1, Relational Operator2/1
  Mod1/1 -> Switch2/3, Switch1/3, Unit Delay/1, Relational Operator/1
  Triggered Subsystem/1(Change Time) -> Add2/2
  Add2/1 -> Relational Operator1/1
  Relational Operator2/1 -> OR/2
  Constant2/1 -> Relational Operator2/2
  OR/1 -> AND/2
  Switch2/1 -> t_leg/1
  Relational Operator3/1 -> Switch2/2
  tdur/1 -> Gain/1, Mod1/2, Relational Operator3/2, Relational Operator1/2
  Add4/1 -> Relational Operator3/1

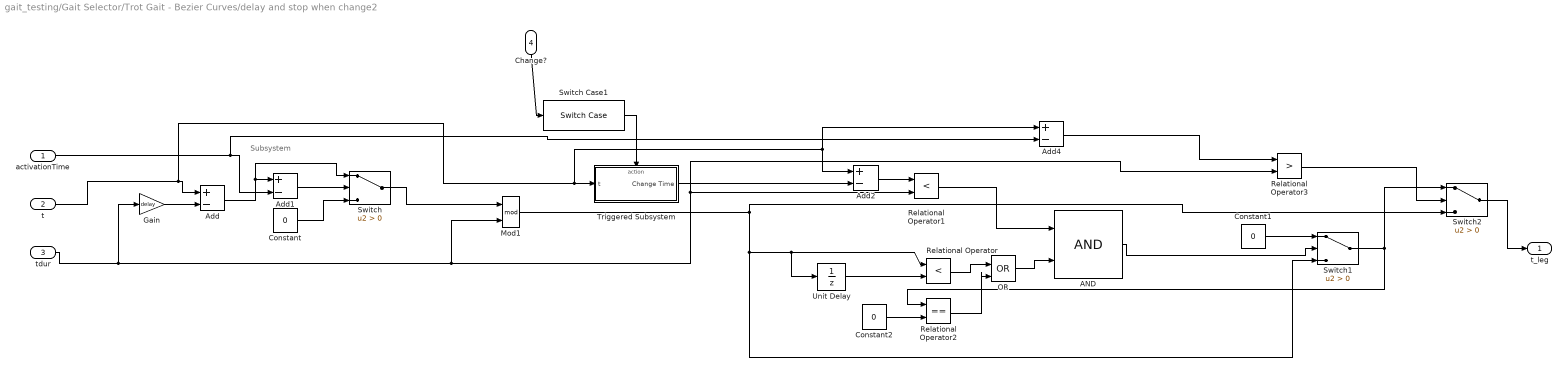
== system gait_testing/Gait Selector/Trot Gait - Bezier Curves/delay and stop when change2 ==
  note: Subsystem
  activationTime : Inport
  t : Inport  Port=2
  tdur : Inport  Port=3
  Change? : Inport  Port=4
  AND : Logic  IconShape=distinctive  AllPortsSameDT=off  OutDataTypeStr=boolean
  Add{,1..2,4} (4 alike) : Sum  Inputs=+-
  Constant : Constant  Value=0
  Constant1 : Constant  Value=0
  Constant2 : Constant  Value=0
  Gain : Gain  Gain=delay
  Mod1 : Math  Operator=mod
  OR : Logic  Operator=OR  IconShape=distinctive  AllPortsSameDT=off  OutDataTypeStr=boolean
  Relational Operator : RelationalOperator  Operator=<  OutDataTypeStr=boolean  RndMeth=Simplest  InputSameDT=off
  Relational Operator1 : RelationalOperator  Operator=<  OutDataTypeStr=boolean  RndMeth=Simplest  InputSameDT=off
  Relational Operator2 : RelationalOperator  Operator===  OutDataTypeStr=boolean  RndMeth=Simplest  InputSameDT=off
  Relational Operator3 : RelationalOperator  Operator=>  OutDataTypeStr=boolean  RndMeth=Simplest  InputSameDT=off
  Switch : Switch  Criteria=u2 > Threshold  SaturateOnIntegerOverflow=off  InputSameDT=off
  Switch Case1 : SwitchCase  ShowDefaultCase=off
  Switch1 : Switch  Criteria=u2 > Threshold  SaturateOnIntegerOverflow=off  InputSameDT=off
  Switch2 : Switch  Criteria=u2 > Threshold  SaturateOnIntegerOverflow=off  InputSameDT=off
  Triggered Subsystem : Subsystem  TreatAsAtomicUnit=on
  Unit Delay : UnitDelay  SampleTime=-1  HasFrameUpgradeWarning=on
  t_leg : Outport
  wires:
  Switch/1 -> Mod1/1
  Gain/1 -> Add/2
  t/1 -> Add2/1, Add4/1, Triggered Subsystem/1(t), Add/1
  Constant/1 -> Switch/3
  Add1/1 -> Switch/2
  activationTime/1 -> Add4/2, Add1/2
  Add/1 -> Switch/1, Add1/1
  Switch Case1/1 -> Triggered Subsystem/Action
  Relational Operator1/1 -> AND/1
  Constant1/1 -> Switch1/1
  Relational Operator/1 -> OR/1
  Change?/1 -> Switch Case1/1
  Unit Delay/1 -> Relational Operator/2
  AND/1 -> Switch1/2
  Switch1/1 -> Switch2/1, Relational Operator2/1
  Mod1/1 -> Switch2/3, Switch1/3, Unit Delay/1, Relational Operator/1
  Triggered Subsystem/1(Change Time) -> Add2/2
  Add2/1 -> Relational Operator1/1
  Relational Operator2/1 -> OR/2
  Constant2/1 -> Relational Operator2/2
  OR/1 -> AND/2
  Switch2/1 -> t_leg/1
  Relational Operator3/1 -> Switch2/2
  tdur/1 -> Gain/1, Mod1/2, Relational Operator3/2, Relational Operator1/2
  Add4/1 -> Relational Operator3/1

== system gait_testing/Gait Selector/Trot Gait - Drive Function/left Back Hip gait ==
  t : Inport
  tdur : Inport  Port=2
  Add : Sum
  Add1 : Sum  Inputs=+++
  Constant : Constant  Value=uMin + (uMax-uMin)/2
  Constant{3,6..8} (4 alike) : Constant  Value=0
  Divide{,1..3} (4 alike) : Product  Inputs=*/
  Gain : Gain  Gain=-1
  Gain1 : Gain  Gain=-1
  Gain2 : Gain  Gain=-1
  Gain5 : Gain  Gain=(uMax-uMin)/2
  If Action Subsystem : Subsystem  TreatAsAtomicUnit=on
  If Action Subsystem1 : Subsystem  TreatAsAtomicUnit=on
  If Action Subsystem2 : Subsystem  TreatAsAtomicUnit=on
  Switch : Switch  Criteria=u2 > Threshold  Threshold=3/8  SaturateOnIntegerOverflow=off  InputSameDT=off
  Switch1 : Switch  Criteria=u2 > Threshold  Threshold=3/8  SaturateOnIntegerOverflow=off  InputSameDT=off
  Switch2 : Switch  Criteria=u2 > Threshold  Threshold=5/8  SaturateOnIntegerOverflow=off  InputSameDT=off
  Switch3 : Switch  Criteria=u2 > Threshold  Threshold=5/8  SaturateOnIntegerOverflow=off  InputSameDT=off
  Out1 : Outport
  wires:
  If Action Subsystem1/1(Out1) -> Switch1/1
  Constant7/1 -> Switch2/1
  Switch1/1 -> Switch2/3
  t/1 -> If Action Subsystem2/1(In1), Divide2/1, Divide1/1, Divide/1, If Action Subsystem1/1(In1), If Action Subsystem/1(In1), Divide3/1
  Add1/1 -> Gain5/1
  If Action Subsystem2/1(Out1) -> Switch3/1
  Switch/1 -> Gain/1
  If Action Subsystem/1(Out1) -> Switch/3
  Constant3/1 -> Switch1/3
  Constant8/1 -> Switch3/3
  Switch3/1 -> Gain2/1
  Switch2/1 -> Gain1/1
  Constant6/1 -> Switch/1
  Gain5/1 -> Add/1
  Constant/1 -> Add/2
  Add/1 -> Out1/1
  Gain/1 -> Add1/3
  Gain1/1 -> Add1/2
  Gain2/1 -> Add1/1
  tdur/1 -> If Action Subsystem/2(tdur), Divide3/2, Divide/2, If Action Subsystem1/2(tdur), If Action Subsystem2/2(tdur), Divide2/2, Divide1/2
  Divide/1 -> Switch1/2
  Divide1/1 -> Switch2/2
  Divide2/1 -> Switch3/2
  Divide3/1 -> Switch/2

== system gait_testing/Gait Selector/Trot Gait - Drive Function/left Back Knee gait ==
  t : Inport
  tdur : Inport  Port=2
  Add : Sum
  Constant : Constant  Value=lMin
  Constant10 : Constant  Value=0
  Constant4 : Constant  Value=0
  Divide : Product  Inputs=*/
  Divide1 : Product  Inputs=*/
  Gain7 : Gain  Gain=-(lMax-lMin)
  If Action Subsystem4 : Subsystem  TreatAsAtomicUnit=on
  Switch5 : Switch  Criteria=u2 > Threshold  Threshold=3/8  SaturateOnIntegerOverflow=off  InputSameDT=off
  Switch6 : Switch  Criteria=u2 > Threshold  Threshold=5/8  SaturateOnIntegerOverflow=off  InputSameDT=off
  Out1 : Outport
  wires:
  If Action Subsystem4/1(Out1) -> Switch5/1
  Switch5/1 -> Switch6/3
  t/1 -> Divide1/1, Divide/1, If Action Subsystem4/1(In1)
  Constant4/1 -> Switch5/3
  Constant10/1 -> Switch6/1
  Switch6/1 -> Gain7/1
  Gain7/1 -> Add/1
  Add/1 -> Out1/1
  Constant/1 -> Add/2
  Divide/1 -> Switch5/2
  tdur/1 -> If Action Subsystem4/2(tdur), Divide1/2, Divide/2
  Divide1/1 -> Switch6/2

== system gait_testing/Gait Selector/Trot Gait - Drive Function/left Front Hip gait ==
  t : Inport
  tdur : Inport  Port=2
  Add : Sum
  Add1 : Sum  Inputs=+++
  Constant : Constant  Value=uMin + (uMax-uMin)/2
  Constant{3,6..8} (4 alike) : Constant  Value=0
  Divide{,1..3} (4 alike) : Product  Inputs=*/
  Gain : Gain  Gain=-1
  Gain1 : Gain  Gain=-1
  Gain2 : Gain  Gain=-1
  Gain5 : Gain  Gain=(uMax-uMin)/2
  If Action Subsystem : Subsystem  TreatAsAtomicUnit=on
  If Action Subsystem1 : Subsystem  TreatAsAtomicUnit=on
  If Action Subsystem2 : Subsystem  TreatAsAtomicUnit=on
  Switch : Switch  Criteria=u2 > Threshold  Threshold=3/8  SaturateOnIntegerOverflow=off  InputSameDT=off
  Switch1 : Switch  Criteria=u2 > Threshold  Threshold=3/8  SaturateOnIntegerOverflow=off  InputSameDT=off
  Switch2 : Switch  Criteria=u2 > Threshold  Threshold=5/8  SaturateOnIntegerOverflow=off  InputSameDT=off
  Switch3 : Switch  Criteria=u2 > Threshold  Threshold=5/8  SaturateOnIntegerOverflow=off  InputSameDT=off
  Out1 : Outport
  wires:
  If Action Subsystem1/1(Out1) -> Switch1/1
  Constant7/1 -> Switch2/1
  Switch1/1 -> Switch2/3
  t/1 -> If Action Subsystem2/1(In1), Divide2/1, Divide1/1, Divide/1, If Action Subsystem1/1(In1), If Action Subsystem/1(In1), Divide3/1
  Add1/1 -> Gain5/1
  If Action Subsystem2/1(Out1) -> Switch3/1
  Switch/1 -> Gain/1
  If Action Subsystem/1(Out1) -> Switch/3
  Constant3/1 -> Switch1/3
  Constant8/1 -> Switch3/3
  Switch3/1 -> Gain2/1
  Switch2/1 -> Gain1/1
  Constant6/1 -> Switch/1
  Gain5/1 -> Add/1
  Constant/1 -> Add/2
  Add/1 -> Out1/1
  Gain/1 -> Add1/3
  Gain1/1 -> Add1/2
  Gain2/1 -> Add1/1
  tdur/1 -> If Action Subsystem/2(tdur), Divide3/2, Divide/2, If Action Subsystem1/2(tdur), If Action Subsystem2/2(tdur), Divide2/2, Divide1/2
  Divide/1 -> Switch1/2
  Divide1/1 -> Switch2/2
  Divide2/1 -> Switch3/2
  Divide3/1 -> Switch/2

== system gait_testing/Gait Selector/Trot Gait - Drive Function/left Front Knee gait ==
  t : Inport
  tdur : Inport  Port=2
  Add : Sum
  Constant : Constant  Value=lMin
  Constant10 : Constant  Value=0
  Constant4 : Constant  Value=0
  Divide : Product  Inputs=*/
  Divide1 : Product  Inputs=*/
  Gain7 : Gain  Gain=-(lMax-lMin)
  If Action Subsystem4 : Subsystem  TreatAsAtomicUnit=on
  Switch5 : Switch  Criteria=u2 > Threshold  Threshold=3/8  SaturateOnIntegerOverflow=off  InputSameDT=off
  Switch6 : Switch  Criteria=u2 > Threshold  Threshold=5/8  SaturateOnIntegerOverflow=off  InputSameDT=off
  Out1 : Outport
  wires:
  If Action Subsystem4/1(Out1) -> Switch5/1
  Switch5/1 -> Switch6/3
  t/1 -> Divide1/1, Divide/1, If Action Subsystem4/1(In1)
  Constant4/1 -> Switch5/3
  Constant10/1 -> Switch6/1
  Switch6/1 -> Gain7/1
  Gain7/1 -> Add/1
  Add/1 -> Out1/1
  Constant/1 -> Add/2
  Divide/1 -> Switch5/2
  tdur/1 -> If Action Subsystem4/2(tdur), Divide1/2, Divide/2
  Divide1/1 -> Switch6/2

== system gait_testing/Gait Selector/Trot Gait - Drive Function/right Back Hip gait ==
  t : Inport
  tdur : Inport  Port=2
  Add : Sum
  Add1 : Sum  Inputs=+++
  Constant : Constant  Value=uMin + (uMax-uMin)/2
  Constant{3,6..8} (4 alike) : Constant  Value=0
  Divide{,1..3} (4 alike) : Product  Inputs=*/
  Gain : Gain  Gain=-1
  Gain1 : Gain  Gain=-1
  Gain2 : Gain  Gain=-1
  Gain5 : Gain  Gain=(uMax-uMin)/2
  If Action Subsystem : Subsystem  TreatAsAtomicUnit=on
  If Action Subsystem1 : Subsystem  TreatAsAtomicUnit=on
  If Action Subsystem2 : Subsystem  TreatAsAtomicUnit=on
  Switch : Switch  Criteria=u2 > Threshold  Threshold=3/8  SaturateOnIntegerOverflow=off  InputSameDT=off
  Switch1 : Switch  Criteria=u2 > Threshold  Threshold=3/8  SaturateOnIntegerOverflow=off  InputSameDT=off
  Switch2 : Switch  Criteria=u2 > Threshold  Threshold=5/8  SaturateOnIntegerOverflow=off  InputSameDT=off
  Switch3 : Switch  Criteria=u2 > Threshold  Threshold=5/8  SaturateOnIntegerOverflow=off  InputSameDT=off
  Out1 : Outport
  wires:
  If Action Subsystem1/1(Out1) -> Switch1/1
  Constant7/1 -> Switch2/1
  Switch1/1 -> Switch2/3
  t/1 -> If Action Subsystem2/1(In1), Divide2/1, Divide1/1, Divide/1, If Action Subsystem1/1(In1), If Action Subsystem/1(In1), Divide3/1
  Add1/1 -> Gain5/1
  If Action Subsystem2/1(Out1) -> Switch3/1
  Switch/1 -> Gain/1
  If Action Subsystem/1(Out1) -> Switch/3
  Constant3/1 -> Switch1/3
  Constant8/1 -> Switch3/3
  Switch3/1 -> Gain2/1
  Switch2/1 -> Gain1/1
  Constant6/1 -> Switch/1
  Gain5/1 -> Add/1
  Constant/1 -> Add/2
  Add/1 -> Out1/1
  Gain/1 -> Add1/3
  Gain1/1 -> Add1/2
  Gain2/1 -> Add1/1
  tdur/1 -> If Action Subsystem/2(tdur), Divide3/2, Divide/2, If Action Subsystem1/2(tdur), If Action Subsystem2/2(tdur), Divide2/2, Divide1/2
  Divide/1 -> Switch1/2
  Divide1/1 -> Switch2/2
  Divide2/1 -> Switch3/2
  Divide3/1 -> Switch/2

== system gait_testing/Gait Selector/Trot Gait - Drive Function/right Back Knee gait ==
  t : Inport
  tdur : Inport  Port=2
  Add : Sum
  Constant : Constant  Value=lMin
  Constant10 : Constant  Value=0
  Constant4 : Constant  Value=0
  Divide : Product  Inputs=*/
  Divide1 : Product  Inputs=*/
  Gain7 : Gain  Gain=-(lMax-lMin)
  If Action Subsystem4 : Subsystem  TreatAsAtomicUnit=on
  Switch5 : Switch  Criteria=u2 > Threshold  Threshold=3/8  SaturateOnIntegerOverflow=off  InputSameDT=off
  Switch6 : Switch  Criteria=u2 > Threshold  Threshold=5/8  SaturateOnIntegerOverflow=off  InputSameDT=off
  Out1 : Outport
  wires:
  If Action Subsystem4/1(Out1) -> Switch5/1
  Switch5/1 -> Switch6/3
  t/1 -> Divide1/1, Divide/1, If Action Subsystem4/1(In1)
  Constant4/1 -> Switch5/3
  Constant10/1 -> Switch6/1
  Switch6/1 -> Gain7/1
  Gain7/1 -> Add/1
  Add/1 -> Out1/1
  Constant/1 -> Add/2
  Divide/1 -> Switch5/2
  tdur/1 -> If Action Subsystem4/2(tdur), Divide1/2, Divide/2
  Divide1/1 -> Switch6/2

== system gait_testing/Gait Selector/Trot Gait - Drive Function/right Front Hip gait ==
  t : Inport
  tdur : Inport  Port=2
  Add : Sum
  Add1 : Sum  Inputs=+++
  Constant : Constant  Value=uMin + (uMax-uMin)/2
  Constant{3,6..8} (4 alike) : Constant  Value=0
  Divide{,1..3} (4 alike) : Product  Inputs=*/
  Gain : Gain  Gain=-1
  Gain1 : Gain  Gain=-1
  Gain2 : Gain  Gain=-1
  Gain5 : Gain  Gain=(uMax-uMin)/2
  If Action Subsystem : Subsystem  TreatAsAtomicUnit=on
  If Action Subsystem1 : Subsystem  TreatAsAtomicUnit=on
  If Action Subsystem2 : Subsystem  TreatAsAtomicUnit=on
  Switch : Switch  Criteria=u2 > Threshold  Threshold=3/8  SaturateOnIntegerOverflow=off  InputSameDT=off
  Switch1 : Switch  Criteria=u2 > Threshold  Threshold=3/8  SaturateOnIntegerOverflow=off  InputSameDT=off
  Switch2 : Switch  Criteria=u2 > Threshold  Threshold=5/8  SaturateOnIntegerOverflow=off  InputSameDT=off
  Switch3 : Switch  Criteria=u2 > Threshold  Threshold=5/8  SaturateOnIntegerOverflow=off  InputSameDT=off
  Out1 : Outport
  wires:
  If Action Subsystem1/1(Out1) -> Switch1/1
  Constant7/1 -> Switch2/1
  Switch1/1 -> Switch2/3
  t/1 -> If Action Subsystem2/1(In1), Divide2/1, Divide1/1, Divide/1, If Action Subsystem1/1(In1), If Action Subsystem/1(In1), Divide3/1
  Add1/1 -> Gain5/1
  If Action Subsystem2/1(Out1) -> Switch3/1
  Switch/1 -> Gain/1
  If Action Subsystem/1(Out1) -> Switch/3
  Constant3/1 -> Switch1/3
  Constant8/1 -> Switch3/3
  Switch3/1 -> Gain2/1
  Switch2/1 -> Gain1/1
  Constant6/1 -> Switch/1
  Gain5/1 -> Add/1
  Constant/1 -> Add/2
  Add/1 -> Out1/1
  Gain/1 -> Add1/3
  Gain1/1 -> Add1/2
  Gain2/1 -> Add1/1
  tdur/1 -> If Action Subsystem/2(tdur), Divide3/2, Divide/2, If Action Subsystem1/2(tdur), If Action Subsystem2/2(tdur), Divide2/2, Divide1/2
  Divide/1 -> Switch1/2
  Divide1/1 -> Switch2/2
  Divide2/1 -> Switch3/2
  Divide3/1 -> Switch/2

== system gait_testing/Gait Selector/Trot Gait - Drive Function/right Front Knee gait ==
  t : Inport
  tdur : Inport  Port=2
  Add : Sum
  Constant : Constant  Value=lMin
  Constant10 : Constant  Value=0
  Constant4 : Constant  Value=0
  Divide : Product  Inputs=*/
  Divide1 : Product  Inputs=*/
  Gain7 : Gain  Gain=-(lMax-lMin)
  If Action Subsystem4 : Subsystem  TreatAsAtomicUnit=on
  Switch5 : Switch  Criteria=u2 > Threshold  Threshold=3/8  SaturateOnIntegerOverflow=off  InputSameDT=off
  Switch6 : Switch  Criteria=u2 > Threshold  Threshold=5/8  SaturateOnIntegerOverflow=off  InputSameDT=off
  Out1 : Outport
  wires:
  If Action Subsystem4/1(Out1) -> Switch5/1
  Switch5/1 -> Switch6/3
  t/1 -> Divide1/1, Divide/1, If Action Subsystem4/1(In1)
  Constant4/1 -> Switch5/3
  Constant10/1 -> Switch6/1
  Switch6/1 -> Gain7/1
  Gain7/1 -> Add/1
  Add/1 -> Out1/1
  Constant/1 -> Add/2
  Divide/1 -> Switch5/2
  tdur/1 -> If Action Subsystem4/2(tdur), Divide1/2, Divide/2
  Divide1/1 -> Switch6/2
